simulink subsystem "H175_cathode"  (R2022b)
settings: Solver=VariableStepAuto  StartTime=0.0  StopTime=10.0  RelTol=1e-3
libraries: fl_lib x88, nesl_utility x73, SimscapeFluids_lib x10, slpidlib x2, BraytonCycle_lib x2
(part 1 of 4)
settings Model: Creator=adrian.taveras  LastModifiedBy=adrian.taveras

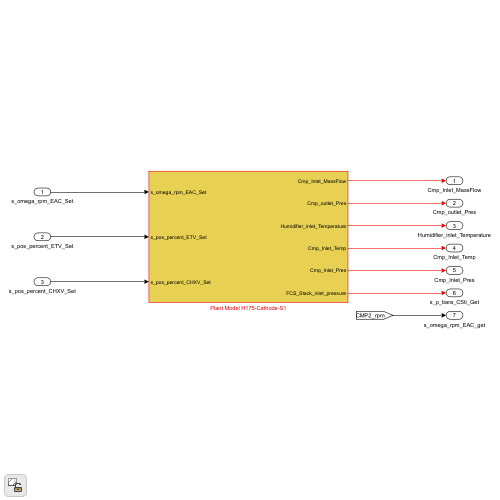
[thumbnail: Simulink's stored preview of the top-level diagram]
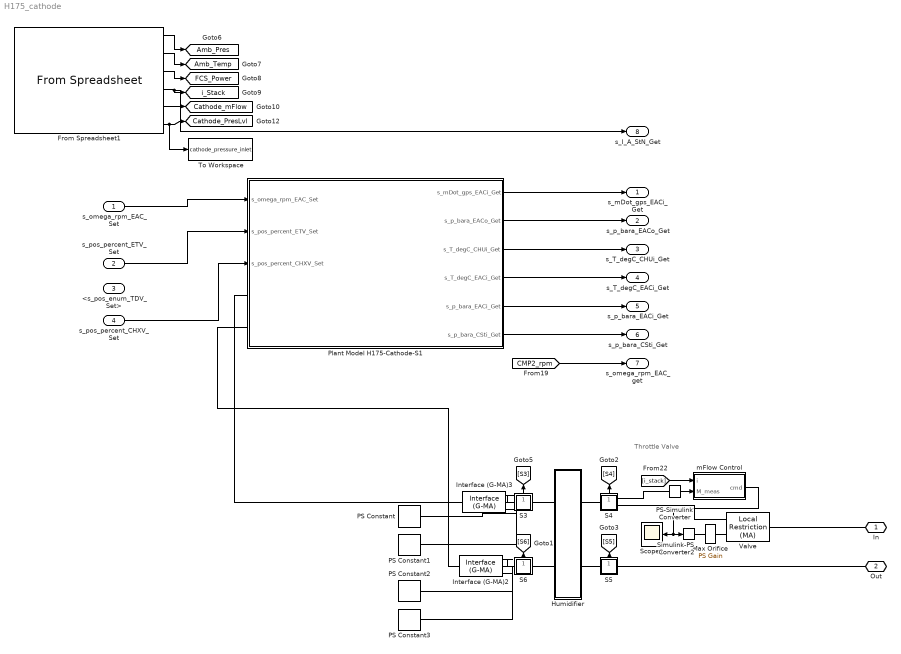
== system H175_cathode ==
  note: Throttle Valve
  s_omega_rpm_EAC_Set : Inport
  s_pos_percent_ETV_Set : Inport  Port=2
  <s_pos_enum_TDV_Set> : Inport  Port=3
  s_pos_percent_CHXV_Set : Inport  Port=4
  From Spreadsheet1 : FromSpreadsheet  FileName=C:\Users\adrian.taveras\Desktop\04-H175-Cathode\H175_Cathode_variables.xlsx  Range=A2:G15
  Humidifier : Subsystem
  Interface (G-MA)2 : SimscapeFluids_lib/Fluid Network Interfaces/Interface (G-MA)  interface_type=foundation.enum.constant_controlled.controlled  moisture_spec=foundation.enum.moisture_spec.relative_humidity  RH_interface=0.5  x_w_interface=0.01  y_w_interface=0.01  HR_interface=0.01  trace_gas_spec=foundation.enum.trace_gas_spec.mass_fraction  x_g_interface=1  y_g_interface=0.001  RH_ws=1  area=0.01 m^2  input_error_spec=foundation.enum.input_range_error.warn
      settings: InternalSimscapePortConfiguration="{\"Bottom\":[{\"id\":\"W\",\"label\":\"W\",\"type\":\"input\"},{\"id\":\"TG\",\"label\":\"TG\",\"type\":\"input\"}],\"Left\":[{\"id\":\"G\",\"label\":\"G\",\"type\":\"foundation.gas.gas\"}],\"Right\":[{\"id\":\"MA\",\"label\":\"MA\",\"type\":\"foundation.moist_air.moist_air\"}],\"Top\":[]}"
  Interface (G-MA)3 : SimscapeFluids_lib/Fluid Network Interfaces/Interface (G-MA)  interface_type=foundation.enum.constant_controlled.controlled  moisture_spec=foundation.enum.moisture_spec.relative_humidity  RH_interface=0.5  x_w_interface=0.01  y_w_interface=0.01  HR_interface=0.01  trace_gas_spec=foundation.enum.trace_gas_spec.mass_fraction  x_g_interface=1  y_g_interface=0.001  RH_ws=1  area=0.01 m^2  input_error_spec=foundation.enum.input_range_error.warn
      settings: InternalSimscapePortConfiguration="{\"Bottom\":[{\"id\":\"W\",\"label\":\"W\",\"type\":\"input\"},{\"id\":\"TG\",\"label\":\"TG\",\"type\":\"input\"}],\"Left\":[{\"id\":\"G\",\"label\":\"G\",\"type\":\"foundation.gas.gas\"}],\"Right\":[{\"id\":\"MA\",\"label\":\"MA\",\"type\":\"foundation.moist_air.moist_air\"}],\"Top\":[]}"
  Max Orifice : fl_lib/Physical Signals/Functions/PS Gain  gain=.008 m^2
  PS Constant : fl_lib/Physical Signals/Sources/PS Constant  constant=.5
  PS Constant1 : fl_lib/Physical Signals/Sources/PS Constant  constant=.001
  PS Constant2 : fl_lib/Physical Signals/Sources/PS Constant  constant=.88
  PS Constant3 : fl_lib/Physical Signals/Sources/PS Constant  constant=.01
  PS-Simulink Converter : nesl_utility/PS-Simulink Converter  PhysicalDomain=network_engine_domain  SubClassName=ps_output  LeftPortType=input  RightPortType=output  PseudoPeriodic=off  Frequencies=[]  VectorFormat=inherit  Unit=inherit  AffineConversion=off
  Plant Model H175-Cathode-S1 : Subsystem
  S3 : Subsystem
      settings: PortSchema="{\"entries\":[{\"content\":{\"sides\":[{\"content\":{\"connectorIds\":[\"LConn1\"]},\"type\":\"ConnectorPlacement.EquallySpacedRectSide\",\"uuid\":\"254e2835-1051-41ce-ae2c-1054ced4b7e5\"},{\"content\":{\"connectorIds\":[\"RConn1\"],\"side\":\"RIGHT\"},\"type\":\"ConnectorPlacement.EquallySpacedRectSide\",\"uuid\":\"319e61c8-525d-4586-8cb8-060a189dde36\"},{\"content\":{\"connectorIds\":[\"Out1\"],\"side\":\"TOP\"},\"type\":\"ConnectorPlacement.EquallySpacedRectSide\",\"uuid\":\"621e15c0-a15c-4528-a2f1-5cf6f15ed99c\"}]},\"type\":\"ConnectorPlacement.EquallySpacedConnector\",\"uuid\":\"0cef8054-f5e2-4319-9020-84a4d4054be4\"}],\"packageUris\":[\"http://schema.mathworks.com/mf0/Connector/R2020b\"],\"version\":\"1.0\"}"
  S4 : Subsystem
      settings: PortSchema="{\"entries\":[{\"content\":{\"sides\":[{\"content\":{\"connectorIds\":[\"LConn1\",\"LConn2\"]},\"type\":\"ConnectorPlacement.EquallySpacedRectSide\",\"uuid\":\"254e2835-1051-41ce-ae2c-1054ced4b7e5\"},{\"content\":{\"connectorIds\":[\"RConn1\"],\"side\":\"RIGHT\"},\"type\":\"ConnectorPlacement.EquallySpacedRectSide\",\"uuid\":\"319e61c8-525d-4586-8cb8-060a189dde36\"},{\"content\":{\"connectorIds\":[\"Out1\"],\"side\":\"TOP\"},\"type\":\"ConnectorPlacement.EquallySpacedRectSide\",\"uuid\":\"621e15c0-a15c-4528-a2f1-5cf6f15ed99c\"}]},\"type\":\"ConnectorPlacement.EquallySpacedConnector\",\"uuid\":\"0cef8054-f5e2-4319-9020-84a4d4054be4\"}],\"packageUris\":[\"http://schema.mathworks.com/mf0/Connector/R2020b\"],\"version\":\"1.0\"}"
  S5 : Subsystem
      settings: PortSchema="{\"entries\":[{\"content\":{\"sides\":[{\"content\":{\"connectorIds\":[\"LConn1\"]},\"type\":\"ConnectorPlacement.EquallySpacedRectSide\",\"uuid\":\"254e2835-1051-41ce-ae2c-1054ced4b7e5\"},{\"content\":{\"connectorIds\":[\"RConn1\"],\"side\":\"RIGHT\"},\"type\":\"ConnectorPlacement.EquallySpacedRectSide\",\"uuid\":\"319e61c8-525d-4586-8cb8-060a189dde36\"},{\"content\":{\"connectorIds\":[\"Out1\"],\"side\":\"TOP\"},\"type\":\"ConnectorPlacement.EquallySpacedRectSide\",\"uuid\":\"621e15c0-a15c-4528-a2f1-5cf6f15ed99c\"},{\"content\":{\"side\":\"BOTTOM\"},\"type\":\"ConnectorPlacement.EquallySpacedRectSide\",\"uuid\":\"5b55ac88-a391-4d8d-b3a5-d7682694097d\"}]},\"type\":\"ConnectorPlacement.EquallySpacedConnector\",\"uuid\":\"0cef8054-f5e2-4319-9020-84a4d4054be4\"}],\"packageUris\":[\"http://schema.mathworks.com/mf0/Connector/R2020b\"],\"version\":\"1.0\"}"
  S6 : Subsystem
      settings: PortSchema="{\"entries\":[{\"content\":{\"sides\":[{\"content\":{\"connectorIds\":[\"LConn1\"]},\"type\":\"ConnectorPlacement.EquallySpacedRectSide\",\"uuid\":\"254e2835-1051-41ce-ae2c-1054ced4b7e5\"},{\"content\":{\"connectorIds\":[\"RConn1\"],\"side\":\"RIGHT\"},\"type\":\"ConnectorPlacement.EquallySpacedRectSide\",\"uuid\":\"319e61c8-525d-4586-8cb8-060a189dde36\"},{\"content\":{\"connectorIds\":[\"Out1\"],\"side\":\"TOP\"},\"type\":\"ConnectorPlacement.EquallySpacedRectSide\",\"uuid\":\"621e15c0-a15c-4528-a2f1-5cf6f15ed99c\"}]},\"type\":\"ConnectorPlacement.EquallySpacedConnector\",\"uuid\":\"0cef8054-f5e2-4319-9020-84a4d4054be4\"}],\"packageUris\":[\"http://schema.mathworks.com/mf0/Connector/R2020b\"],\"version\":\"1.0\"}"
  Scope1 : Scope
  Simulink-PS Converter2 : nesl_utility/Simulink-PS Converter  PhysicalDomain=network_engine_domain  SubClassName=ps_input  LeftPortType=input  RightPortType=output  PseudoPeriodic=off  Frequencies=[]  NoiseDistribution=none  NoiseParameters=[]  Unit=1  AffineConversion=off  FilteringAndDerivatives=filter  SimscapeFilterOrder=1  InputFilterTimeConstant=0.001  UdotUserProvided=0
  To Workspace : ToWorkspace  VariableName=cathode_pressure_inlet  SaveFormat=Timeseries  SampleTime=-1
  Valve : fl_lib/Moist Air/Elements/Local Restriction (MA)  restriction_type=foundation.enum.restriction_type.variable  restriction_area=0.001 m^2  min_area=2e-11 m^2  max_area=.006 m^2  area=.01 m^2  Cd=.64  B_lam=0.999
  mFlow Control : Subsystem
  In : PMIOPort  Side=Left
  Out : PMIOPort  Port=2  Side=Left
  s_mDot_gps_EACi_Get : Outport
  s_p_bara_EACo_Get : Outport  Port=2
  s_T_degC_CHUi_Get : Outport  Port=3
  s_T_degC_EACi_Get : Outport  Port=4
  s_p_bara_EACi_Get : Outport  Port=5
  s_p_bara_CSti_Get : Outport  Port=6
  s_omega_rpm_EAC_get : Outport  Port=7
  s_I_A_StN_Get : Outport  Port=8
  tag scope: Amb_Pres=global, Amb_Temp=global, Cathode_PresLvl=global, Cathode_mFlow=global, FCS_Power=global, i_Stack=global
  wires:
  Plant Model H175-Cathode-S1/3(s_T_degC_CHUi_Get) -> s_T_degC_CHUi_Get/1
  Plant Model H175-Cathode-S1/1(s_mDot_gps_EACi_Get) -> s_mDot_gps_EACi_Get/1
  Plant Model H175-Cathode-S1/2(s_p_bara_EACo_Get) -> s_p_bara_EACo_Get/1
  Plant Model H175-Cathode-S1/4(s_T_degC_EACi_Get) -> s_T_degC_EACi_Get/1
  Plant Model H175-Cathode-S1/5(s_p_bara_EACi_Get) -> s_p_bara_EACi_Get/1
  Plant Model H175-Cathode-S1/6(s_p_bara_CSti_Get) -> s_p_bara_CSti_Get/1
  s_omega_rpm_EAC_Set/1 -> Plant Model H175-Cathode-S1/1(s_omega_rpm_EAC_Set)
  [CMP2_rpm] -> s_omega_rpm_EAC_get/1
  s_pos_percent_ETV_Set/1 -> Plant Model H175-Cathode-S1/2(s_pos_percent_ETV_Set)
  s_pos_percent_CHXV_Set/1 -> Plant Model H175-Cathode-S1/3(s_pos_percent_CHXV_Set)
  From Spreadsheet1/2 -> [Amb_Temp]
  From Spreadsheet1/6 -> [Cathode_PresLvl], To Workspace/1
  From Spreadsheet1/3 -> [FCS_Power]
  From Spreadsheet1/4 -> [i_Stack], s_I_A_StN_Get/1
  From Spreadsheet1/5 -> [Cathode_mFlow]
  From Spreadsheet1/1 -> [Amb_Pres]
  S6/1(Outport) -> [S6]
  S3/1(Outport) -> [S3]
  [i_stack] -> mFlow Control/1(i)
  PS-Simulink Converter/1 -> mFlow Control/2(M_meas)
  mFlow Control/1(cmd) -> Scope1/1, Simulink-PS Converter2/1
  S5/1(Outport) -> [S5]
  S4/1(Outport) -> [S4]
  connections:
  S5/RConn1 -- Humidifier/LConn2
  S3/LConn1 -- Humidifier/RConn1
  Interface (G-MA)3/LConn1 -- Plant Model H175-Cathode-S1/LConn1
  S4/RConn1 -- Humidifier/LConn1
  S4/LConn2 -- Valve/LConn1
  Out/RConn1 -- S5/LConn1
  Simulink-PS Converter2/RConn1 -- Max Orifice/LConn1
  Max Orifice/RConn1 -- Valve/LConn2
  S4/LConn1 -- PS-Simulink Converter/LConn1
  Interface (G-MA)2/RConn1 -- S6/RConn1
  Interface (G-MA)2/LConn1 -- Plant Model H175-Cathode-S1/LConn2
  Valve/RConn1 -- In/RConn1
  Humidifier/RConn2 -- S6/LConn1
  Interface (G-MA)3/RConn1 -- S3/RConn1
  Interface (G-MA)3/RConn2 -- PS Constant/RConn1
  Interface (G-MA)3/RConn3 -- PS Constant1/RConn1
  Interface (G-MA)2/RConn2 -- PS Constant2/RConn1
  Interface (G-MA)2/RConn3 -- PS Constant3/RConn1

== system H175_cathode/Humidifier ==
  Cathode Humidifier1 : Subsystem  Tag=PublishSubsystem
  Cathode Humidifier2 : Subsystem  Tag=PublishSubsystem
  B : PMIOPort  Side=Left
  A1 : PMIOPort  Port=2  Side=Left
  A : PMIOPort  Port=3  Side=Right
  B1 : PMIOPort  Port=4  Side=Right
  connections:
  A1/RConn1 -- Cathode Humidifier2/RConn1
  B/RConn1 -- Cathode Humidifier1/LConn1
  Cathode Humidifier2/LConn1 -- B1/RConn1
  A/RConn1 -- Cathode Humidifier1/RConn1

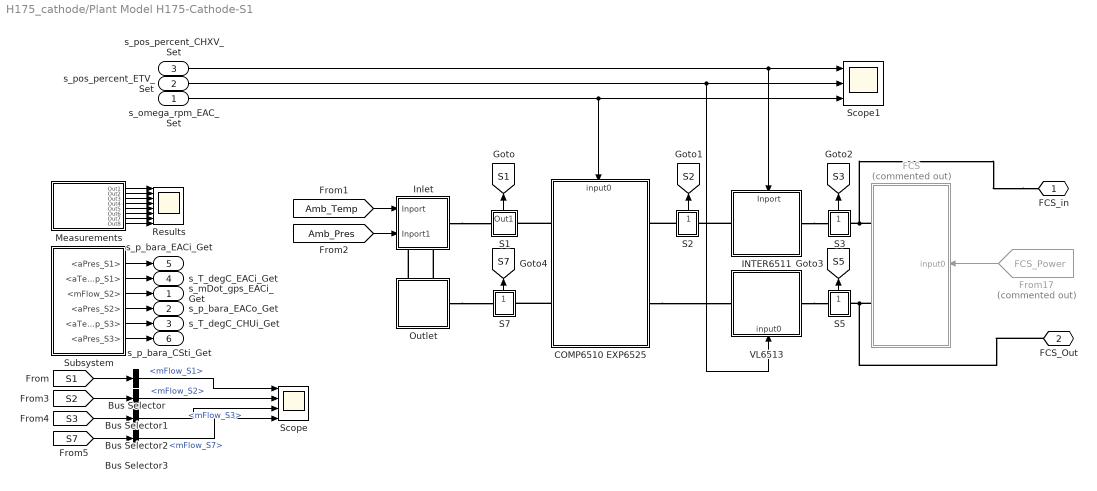
== system H175_cathode/Plant Model H175-Cathode-S1 ==
  s_omega_rpm_EAC_Set : Inport
  s_pos_percent_ETV_Set : Inport  Port=2
  s_pos_percent_CHXV_Set : Inport  Port=3
  "  INTER6511" : Subsystem
      settings: PortSchema="{\"entries\":[{\"content\":{\"sides\":[{\"content\":{\"connectorIds\":[\"LConn1\"]},\"type\":\"ConnectorPlacement.EquallySpacedRectSide\",\"uuid\":\"aadd5cae-df0a-4bff-a962-f45a16973fea\"},{\"content\":{\"connectorIds\":[\"RConn1\"],\"side\":\"RIGHT\"},\"type\":\"ConnectorPlacement.EquallySpacedRectSide\",\"uuid\":\"1cb17e32-c83b-4a61-86cd-0928b2990d84\"},{\"content\":{\"connectorIds\":[\"In1\"],\"side\":\"TOP\"},\"type\":\"ConnectorPlacement.EquallySpacedRectSide\",\"uuid\":\"6373b90c-60a5-4bfd-bcd0-a65342ff5e9d\"}]},\"type\":\"ConnectorPlacement.EquallySpacedConnector\",\"uuid\":\"e3bee535-890d-4344-8b9d-df6658dbcf92\"}],\"packageUris\":[\"http://schema.mathworks.com/mf0/Connector/R2020b\"],\"version\":\"1.0\"}"
  Bus Selector : BusSelector  OutputSignals=mFlow_S1
  Bus Selector1 : BusSelector  OutputSignals=mFlow_S2
  Bus Selector2 : BusSelector  OutputSignals=mFlow_S3
  Bus Selector3 : BusSelector  OutputSignals=mFlow_S7
  COMP6510 EXP6525 : Subsystem
      settings: PortSchema="{\"entries\":[{\"content\":{\"sides\":[{\"content\":{\"connectorIds\":[\"LConn1\",\"LConn2\"]},\"type\":\"ConnectorPlacement.EquallySpacedRectSide\",\"uuid\":\"3b5e743a-f9ab-48a6-a95a-34d49360e365\"},{\"content\":{\"connectorIds\":[\"RConn1\",\"RConn2\"],\"side\":\"RIGHT\"},\"type\":\"ConnectorPlacement.EquallySpacedRectSide\",\"uuid\":\"4725ff20-2386-47e2-9079-da214be67dc0\"},{\"content\":{\"connectorIds\":[\"In1\"],\"side\":\"TOP\"},\"type\":\"ConnectorPlacement.EquallySpacedRectSide\",\"uuid\":\"6967643a-4f8b-418b-b9c8-3e43650ed8fb\"}]},\"type\":\"ConnectorPlacement.EquallySpacedConnector\",\"uuid\":\"78531208-dad3-4e1a-9fde-a0a5eb2a424d\"}],\"packageUris\":[\"http://schema.mathworks.com/mf0/Connector/R2020b\"],\"version\":\"1.0\"}"
  FCS : Subsystem  Commented=on
      settings: PortSchema="{\"entries\":[{\"content\":{\"sides\":[{\"content\":{\"connectorIds\":[\"LConn1\",\"LConn2\"]},\"type\":\"ConnectorPlacement.EquallySpacedRectSide\",\"uuid\":\"2b4fa60d-bbb2-4344-a190-bd8fb686e197\"},{\"content\":{\"connectorIds\":[\"In1\"],\"side\":\"RIGHT\"},\"type\":\"ConnectorPlacement.EquallySpacedRectSide\",\"uuid\":\"0d0ce5e9-3383-4311-ac80-7f18e4d53921\"},{\"content\":{\"connectorIds\":[],\"side\":\"TOP\"},\"type\":\"ConnectorPlacement.EquallySpacedRectSide\",\"uuid\":\"894db579-cef2-48df-a3cf-b374864ac750\"}]},\"type\":\"ConnectorPlacement.EquallySpacedConnector\",\"uuid\":\"d963d44c-ade5-424e-b8d1-081ccbb81476\"}],\"packageUris\":[\"http://schema.mathworks.com/mf0/Connector/R2020b\"],\"version\":\"1.0\"}"
  From17 : From  Commented=on  GotoTag=FCS_Power  TagVisibility=global
  Inlet : Subsystem
      settings: PortSchema="{\"entries\":[{\"content\":{\"sides\":[{\"content\":{\"connectorIds\":[\"In1\",\"In2\"]},\"type\":\"ConnectorPlacement.EquallySpacedRectSide\",\"uuid\":\"383c8b90-d22b-483c-be09-d78d9bde0881\"},{\"content\":{\"connectorIds\":[\"RConn1\"],\"side\":\"RIGHT\"},\"type\":\"ConnectorPlacement.EquallySpacedRectSide\",\"uuid\":\"3dc3e004-4331-4c40-8051-329aa9250422\"},{\"content\":{\"side\":\"TOP\"},\"type\":\"ConnectorPlacement.EquallySpacedRectSide\",\"uuid\":\"aff35d8f-ac03-451a-b72e-dc7bd89924e8\"},{\"content\":{\"connectorIds\":[\"RConn2\",\"RConn3\"],\"side\":\"BOTTOM\"},\"type\":\"ConnectorPlacement.EquallySpacedRectSide\",\"uuid\":\"82493911-a5c4-468a-a003-983b92ffd105\"}]},\"type\":\"ConnectorPlacement.EquallySpacedConnector\",\"uuid\":\"d9a1e9aa-22f5-4e42-bf15-8a8ecd9f58f9\"}],\"packageUris\":[\"http://schema.mathworks.com/mf0/Connector/R2020b\"],\"version\":\"1.0\"}"
  Measurements : Subsystem
  Outlet : Subsystem
      settings: PortSchema="{\"entries\":[{\"content\":{\"sides\":[{\"content\":{\"connectorIds\":[]},\"type\":\"ConnectorPlacement.EquallySpacedRectSide\",\"uuid\":\"36868ebe-cd3e-431e-8c92-72eff994fdca\"},{\"content\":{\"connectorIds\":[\"RConn1\"],\"side\":\"RIGHT\"},\"type\":\"ConnectorPlacement.EquallySpacedRectSide\",\"uuid\":\"888b4745-0282-499a-ac24-9932e912f806\"},{\"content\":{\"connectorIds\":[\"LConn1\",\"LConn2\"],\"side\":\"TOP\"},\"type\":\"ConnectorPlacement.EquallySpacedRectSide\",\"uuid\":\"c9640cda-325e-4343-a4ee-57b72cddf09b\"}]},\"type\":\"ConnectorPlacement.EquallySpacedConnector\",\"uuid\":\"8844a185-194b-4897-895e-d4ee7951df66\"}],\"packageUris\":[\"http://schema.mathworks.com/mf0/Connector/R2020b\"],\"version\":\"1.0\"}"
  Results : Scope  NumInputPorts=8
  S1 : Subsystem
      settings: PortSchema="{\"entries\":[{\"content\":{\"sides\":[{\"content\":{\"connectorIds\":[\"LConn1\"]},\"type\":\"ConnectorPlacement.EquallySpacedRectSide\",\"uuid\":\"872c3fc9-10e2-440a-866c-17ec3b229dcc\"},{\"content\":{\"connectorIds\":[\"RConn1\"],\"side\":\"RIGHT\"},\"type\":\"ConnectorPlacement.EquallySpacedRectSide\",\"uuid\":\"5792e744-d6fd-4953-8a6b-3bc8a25af09f\"},{\"content\":{\"connectorIds\":[\"Out1\"],\"side\":\"TOP\"},\"type\":\"ConnectorPlacement.EquallySpacedRectSide\",\"uuid\":\"2a1362d0-5fde-44c4-8ae5-faebfba0e935\"}]},\"type\":\"ConnectorPlacement.EquallySpacedConnector\",\"uuid\":\"2555ecf8-f6a2-49b2-8cff-d299990cd611\"}],\"packageUris\":[\"http://schema.mathworks.com/mf0/Connector/R2020b\"],\"version\":\"1.0\"}"
  S2 : Subsystem
      settings: PortSchema="{\"entries\":[{\"content\":{\"sides\":[{\"content\":{\"connectorIds\":[\"LConn1\"]},\"type\":\"ConnectorPlacement.EquallySpacedRectSide\",\"uuid\":\"872c3fc9-10e2-440a-866c-17ec3b229dcc\"},{\"content\":{\"connectorIds\":[\"RConn1\"],\"side\":\"RIGHT\"},\"type\":\"ConnectorPlacement.EquallySpacedRectSide\",\"uuid\":\"5792e744-d6fd-4953-8a6b-3bc8a25af09f\"},{\"content\":{\"connectorIds\":[\"Out1\"],\"side\":\"TOP\"},\"type\":\"ConnectorPlacement.EquallySpacedRectSide\",\"uuid\":\"2a1362d0-5fde-44c4-8ae5-faebfba0e935\"}]},\"type\":\"ConnectorPlacement.EquallySpacedConnector\",\"uuid\":\"2555ecf8-f6a2-49b2-8cff-d299990cd611\"}],\"packageUris\":[\"http://schema.mathworks.com/mf0/Connector/R2020b\"],\"version\":\"1.0\"}"
  S3 : Subsystem
      settings: PortSchema="{\"entries\":[{\"content\":{\"sides\":[{\"content\":{\"connectorIds\":[\"LConn1\"]},\"type\":\"ConnectorPlacement.EquallySpacedRectSide\",\"uuid\":\"872c3fc9-10e2-440a-866c-17ec3b229dcc\"},{\"content\":{\"connectorIds\":[\"RConn1\"],\"side\":\"RIGHT\"},\"type\":\"ConnectorPlacement.EquallySpacedRectSide\",\"uuid\":\"5792e744-d6fd-4953-8a6b-3bc8a25af09f\"},{\"content\":{\"connectorIds\":[\"Out1\"],\"side\":\"TOP\"},\"type\":\"ConnectorPlacement.EquallySpacedRectSide\",\"uuid\":\"2a1362d0-5fde-44c4-8ae5-faebfba0e935\"}]},\"type\":\"ConnectorPlacement.EquallySpacedConnector\",\"uuid\":\"2555ecf8-f6a2-49b2-8cff-d299990cd611\"}],\"packageUris\":[\"http://schema.mathworks.com/mf0/Connector/R2020b\"],\"version\":\"1.0\"}"
  S5 : Subsystem
      settings: PortSchema="{\"entries\":[{\"content\":{\"sides\":[{\"content\":{\"connectorIds\":[\"LConn1\"]},\"type\":\"ConnectorPlacement.EquallySpacedRectSide\",\"uuid\":\"872c3fc9-10e2-440a-866c-17ec3b229dcc\"},{\"content\":{\"connectorIds\":[\"RConn1\"],\"side\":\"RIGHT\"},\"type\":\"ConnectorPlacement.EquallySpacedRectSide\",\"uuid\":\"5792e744-d6fd-4953-8a6b-3bc8a25af09f\"},{\"content\":{\"connectorIds\":[\"Out1\"],\"side\":\"TOP\"},\"type\":\"ConnectorPlacement.EquallySpacedRectSide\",\"uuid\":\"2a1362d0-5fde-44c4-8ae5-faebfba0e935\"}]},\"type\":\"ConnectorPlacement.EquallySpacedConnector\",\"uuid\":\"2555ecf8-f6a2-49b2-8cff-d299990cd611\"}],\"packageUris\":[\"http://schema.mathworks.com/mf0/Connector/R2020b\"],\"version\":\"1.0\"}"
  S7 : Subsystem
      settings: PortSchema="{\"entries\":[{\"content\":{\"sides\":[{\"content\":{\"connectorIds\":[\"LConn1\"]},\"type\":\"ConnectorPlacement.EquallySpacedRectSide\",\"uuid\":\"872c3fc9-10e2-440a-866c-17ec3b229dcc\"},{\"content\":{\"connectorIds\":[\"RConn1\"],\"side\":\"RIGHT\"},\"type\":\"ConnectorPlacement.EquallySpacedRectSide\",\"uuid\":\"5792e744-d6fd-4953-8a6b-3bc8a25af09f\"},{\"content\":{\"connectorIds\":[\"Out1\"],\"side\":\"TOP\"},\"type\":\"ConnectorPlacement.EquallySpacedRectSide\",\"uuid\":\"2a1362d0-5fde-44c4-8ae5-faebfba0e935\"}]},\"type\":\"ConnectorPlacement.EquallySpacedConnector\",\"uuid\":\"2555ecf8-f6a2-49b2-8cff-d299990cd611\"}],\"packageUris\":[\"http://schema.mathworks.com/mf0/Connector/R2020b\"],\"version\":\"1.0\"}"
  Scope : Scope  NumInputPorts=4
  Scope1 : Scope  NumInputPorts=3
  Subsystem : Subsystem
  VL6513 : Subsystem
      settings: PortSchema="{\"entries\":[{\"content\":{\"sides\":[{\"content\":{\"connectorIds\":[\"LConn1\"]},\"type\":\"ConnectorPlacement.EquallySpacedRectSide\",\"uuid\":\"aadd5cae-df0a-4bff-a962-f45a16973fea\"},{\"content\":{\"connectorIds\":[\"RConn1\"],\"side\":\"RIGHT\"},\"type\":\"ConnectorPlacement.EquallySpacedRectSide\",\"uuid\":\"1cb17e32-c83b-4a61-86cd-0928b2990d84\"},{\"content\":{\"connectorIds\":[],\"side\":\"TOP\"},\"type\":\"ConnectorPlacement.EquallySpacedRectSide\",\"uuid\":\"6373b90c-60a5-4bfd-bcd0-a65342ff5e9d\"},{\"content\":{\"connectorIds\":[\"In1\"],\"side\":\"BOTTOM\"},\"type\":\"ConnectorPlacement.EquallySpacedRectSide\",\"uuid\":\"d931d881-84c0-4cfd-a67b-0ca607edaec5\"}]},\"type\":\"ConnectorPlacement.EquallySpacedConnector\",\"uuid\":\"e3bee535-890d-4344-8b9d-df6658dbcf92\"}],\"packageUris\":[\"http://schema.mathworks.com/mf0/Connector/R2020b\"],\"version\":\"1.0\"}"
  FCS_in : PMIOPort  Side=Left
  FCS_Out : PMIOPort  Port=2  Side=Left
  s_mDot_gps_EACi_Get : Outport
  s_p_bara_EACo_Get : Outport  Port=2
  s_T_degC_CHUi_Get : Outport  Port=3
  s_T_degC_EACi_Get : Outport  Port=4
  s_p_bara_EACi_Get : Outport  Port=5
  s_p_bara_CSti_Get : Outport  Port=6
  tag scope: S1=global, S2=global, S3=global, S5=global, S7=global
  wires:
  Bus Selector3/1 -> Scope/4  "<mFlow_S7>"
  Bus Selector2/1 -> Scope/3  "<mFlow_S3>"
  Bus Selector1/1 -> Scope/2  "<mFlow_S2>"
  Bus Selector/1 -> Scope/1  "<mFlow_S1>"
  [S7] -> Bus Selector3/1
  [S3] -> Bus Selector2/1
  [S2] -> Bus Selector1/1
  [S1] -> Bus Selector/1
  s_pos_percent_CHXV_Set/1 -> Scope1/1, "  INTER6511"/1(Inport)
  Measurements/8(Out8) -> Results/8
  s_omega_rpm_EAC_Set/1 -> Scope1/3, COMP6510 EXP6525/1(input0)
  Subsystem/4(<aPres_S2>) -> s_p_bara_EACo_Get/1
  Subsystem/2(<aTemp_S1>) -> s_T_degC_EACi_Get/1
  Subsystem/3(<mFlow_S2>) -> s_mDot_gps_EACi_Get/1
  Subsystem/1(<aPres_S1>) -> s_p_bara_EACi_Get/1
  Subsystem/5(<aTemp_S3>) -> s_T_degC_CHUi_Get/1
  Subsystem/6(<aPres_S3>) -> s_p_bara_CSti_Get/1
  S2/1(Out1) -> [S2]
  [Amb_Temp] -> Inlet/1(Inport)
  S7/1(Out1) -> [S7]
  S1/1(Out1) -> [S1]
  [Amb_Pres] -> Inlet/2(Inport1)
  Measurements/6(Out6) -> Results/6
  Measurements/7(Out7) -> Results/7
  Measurements/1(Out1) -> Results/1
  Measurements/3(Out3) -> Results/3
  Measurements/4(Out4) -> Results/4
  Measurements/2(Out2) -> Results/2
  Measurements/5(Out5) -> Results/5
  S3/1(Out1) -> [S3]
  S5/1(Out1) -> [S5]
  s_pos_percent_ETV_Set/1 -> VL6513/1(input0), Scope1/2
  From17/1 -> FCS/1(input0)
  connections:
  COMP6510 EXP6525/RConn2 -- VL6513/LConn1
  COMP6510 EXP6525/LConn2 -- S7/LConn1
  S2/LConn1 -- COMP6510 EXP6525/RConn1
  COMP6510 EXP6525/LConn1 -- S1/RConn1
  "  INTER6511"/LConn1 -- S2/RConn1
  Outlet/LConn2 -- Inlet/RConn3
  Inlet/RConn1 -- S1/LConn1
  Outlet/RConn1 -- S7/RConn1
  Outlet/LConn1 -- Inlet/RConn2
  "  INTER6511"/RConn1 -- S3/RConn1
  FCS_Out/RConn1 -- FCS/LConn2 -- S5/LConn1
  VL6513/RConn1 -- S5/RConn1
  FCS_in/RConn1 -- FCS/LConn1 -- S3/LConn1

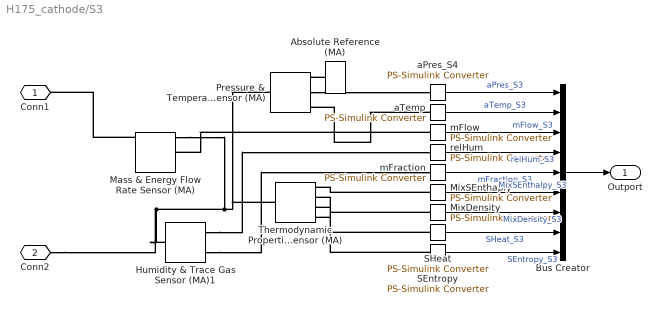
== system H175_cathode/S3 ==
  Absolute Reference (MA) : fl_lib/Moist Air/Elements/Absolute Reference (MA)
  Bus Creator : BusCreator  Inputs=9
  Humidity & Trace Gas Sensor (MA)1 : fl_lib/Moist Air/Sensors/Humidity & Trace Gas Sensor (MA)  moisture_spec=foundation.enum.moisture_spec.relative_humidity  trace_gas_spec=foundation.enum.trace_gas_spec.mass_fraction
      settings: InternalSimscapePortConfiguration="{\"Bottom\":[],\"Left\":[{\"id\":\"A\",\"label\":\"A\",\"type\":\"foundation.moist_air.moist_air\"}],\"Right\":[{\"id\":\"W\",\"label\":\"W\",\"type\":\"output\"},{\"id\":\"G\",\"label\":\"G\",\"type\":\"output\"}],\"Top\":[]}"
  Mass & Energy Flow Rate Sensor (MA) : fl_lib/Moist Air/Sensors/Mass & Energy Flow Rate Sensor (MA)
      settings: InternalSimscapePortConfiguration="{\"Bottom\":[],\"Left\":[{\"id\":\"A\",\"label\":\"A\",\"type\":\"foundation.moist_air.moist_air\"},{\"id\":\"Mw\",\"label\":\"Mw\",\"type\":\"output\"},{\"id\":\"Mg\",\"label\":\"Mg\",\"type\":\"output\"}],\"Right\":[{\"id\":\"B\",\"label\":\"B\",\"type\":\"foundation.moist_air.moist_air\"},{\"id\":\"M\",\"label\":\"M\",\"type\":\"output\"},{\"id\":\"PHI\",\"label\":\"Phi\",\"type\":\"output\"}],\"Top\":[]}"
  MixDensity : nesl_utility/PS-Simulink Converter  PhysicalDomain=network_engine_domain  SubClassName=ps_output  LeftPortType=input  RightPortType=output  PseudoPeriodic=off  Frequencies=[]  VectorFormat=inherit  Unit=inherit  AffineConversion=off
  MixSEnthaply : nesl_utility/PS-Simulink Converter  PhysicalDomain=network_engine_domain  SubClassName=ps_output  LeftPortType=input  RightPortType=output  PseudoPeriodic=off  Frequencies=[]  VectorFormat=inherit  Unit=inherit  AffineConversion=off
  Pressure & Temperature Sensor (MA) : fl_lib/Moist Air/Sensors/Pressure & Temperature Sensor (MA)
      settings: InternalSimscapePortConfiguration="{\"Bottom\":[],\"Left\":[{\"id\":\"A\",\"label\":\"A\",\"type\":\"foundation.moist_air.moist_air\"}],\"Right\":[{\"id\":\"B\",\"label\":\"B\",\"type\":\"foundation.moist_air.moist_air\"},{\"id\":\"P\",\"label\":\"P\",\"type\":\"output\"},{\"id\":\"T\",\"label\":\"T\",\"type\":\"output\"}],\"Top\":[]}"
  SEntropy : nesl_utility/PS-Simulink Converter  PhysicalDomain=network_engine_domain  SubClassName=ps_output  LeftPortType=input  RightPortType=output  PseudoPeriodic=off  Frequencies=[]  VectorFormat=inherit  Unit=inherit  AffineConversion=off
  SHeat : nesl_utility/PS-Simulink Converter  PhysicalDomain=network_engine_domain  SubClassName=ps_output  LeftPortType=input  RightPortType=output  PseudoPeriodic=off  Frequencies=[]  VectorFormat=inherit  Unit=inherit  AffineConversion=off
  Thermodynamic Properties Sensor (MA) : fl_lib/Moist Air/Sensors/Thermodynamic Properties Sensor (MA)  measurement_mass_spec=foundation.enum.measurement_mass_spec.mixture
      settings: InternalSimscapePortConfiguration="{\"Bottom\":[],\"Left\":[{\"id\":\"A\",\"label\":\"A\",\"type\":\"foundation.moist_air.moist_air\"}],\"Right\":[{\"id\":\"H\",\"label\":\"h\",\"type\":\"output\"},{\"id\":\"RHO\",\"label\":\"rho\",\"type\":\"output\"},{\"id\":\"CP\",\"label\":\"cp\",\"type\":\"output\"},{\"id\":\"S\",\"label\":\"s\",\"type\":\"output\"}],\"Top\":[]}"
  aPres_S4 : nesl_utility/PS-Simulink Converter  PhysicalDomain=network_engine_domain  SubClassName=ps_output  LeftPortType=input  RightPortType=output  PseudoPeriodic=off  Frequencies=[]  VectorFormat=inherit  Unit=inherit  AffineConversion=off
  aTemp : nesl_utility/PS-Simulink Converter  PhysicalDomain=network_engine_domain  SubClassName=ps_output  LeftPortType=input  RightPortType=output  PseudoPeriodic=off  Frequencies=[]  VectorFormat=inherit  Unit=inherit  AffineConversion=off
  mFlow : nesl_utility/PS-Simulink Converter  PhysicalDomain=network_engine_domain  SubClassName=ps_output  LeftPortType=input  RightPortType=output  PseudoPeriodic=off  Frequencies=[]  VectorFormat=inherit  Unit=inherit  AffineConversion=off
  mFraction : nesl_utility/PS-Simulink Converter  PhysicalDomain=network_engine_domain  SubClassName=ps_output  LeftPortType=input  RightPortType=output  PseudoPeriodic=off  Frequencies=[]  VectorFormat=inherit  Unit=inherit  AffineConversion=off
  relHum : nesl_utility/PS-Simulink Converter  PhysicalDomain=network_engine_domain  SubClassName=ps_output  LeftPortType=input  RightPortType=output  PseudoPeriodic=off  Frequencies=[]  VectorFormat=inherit  Unit=inherit  AffineConversion=off
  Conn1 : PMIOPort  Side=Left
  Conn2 : PMIOPort  Port=2  Side=Right
  Outport : Outport
  wires:
  SHeat/1 -> Bus Creator/8  "SHeat_S3"
  Bus Creator/1 -> Outport/1
  relHum/1 -> Bus Creator/4  "relHum_S3"
  mFlow/1 -> Bus Creator/3  "mFlow_S3"
  mFraction/1 -> Bus Creator/5  "mFraction_S3"
  MixDensity/1 -> Bus Creator/7  "MixDensity_S3"
  MixSEnthaply/1 -> Bus Creator/6  "MixSEnthalpy_S3"
  SEntropy/1 -> Bus Creator/9  "SEntropy_S3"
  aPres_S4/1 -> Bus Creator/1  "aPres_S3"
  aTemp/1 -> Bus Creator/2  "aTemp_S3"
  connections:
  Absolute Reference (MA)/LConn1 -- Pressure & Temperature Sensor (MA)/RConn1
  Humidity & Trace Gas Sensor (MA)1/RConn2 -- mFraction/LConn1
  Pressure & Temperature Sensor (MA)/RConn2 -- aPres_S4/LConn1
  mFlow/LConn1 -- Mass & Energy Flow Rate Sensor (MA)/RConn2
  Humidity & Trace Gas Sensor (MA)1/LConn1 -- Pressure & Temperature Sensor (MA)/LConn1 -- Thermodynamic Properties Sensor (MA)/LConn1 -- Mass & Energy Flow Rate Sensor (MA)/RConn1 -- Conn2/RConn1
  SEntropy/LConn1 -- Thermodynamic Properties Sensor (MA)/RConn3
  aTemp/LConn1 -- Pressure & Temperature Sensor (MA)/RConn3
  SHeat/LConn1 -- Thermodynamic Properties Sensor (MA)/RConn4
  MixDensity/LConn1 -- Thermodynamic Properties Sensor (MA)/RConn2
  MixSEnthaply/LConn1 -- Thermodynamic Properties Sensor (MA)/RConn1
  Humidity & Trace Gas Sensor (MA)1/RConn1 -- relHum/LConn1
  Mass & Energy Flow Rate Sensor (MA)/LConn1 -- Conn1/RConn1

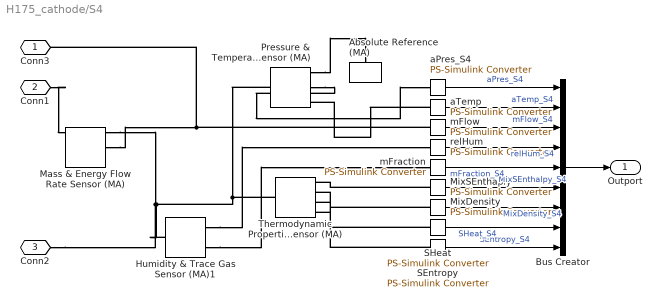
== system H175_cathode/S4 ==
  Absolute Reference (MA) : fl_lib/Moist Air/Elements/Absolute Reference (MA)
  Bus Creator : BusCreator  Inputs=9
  Humidity & Trace Gas Sensor (MA)1 : fl_lib/Moist Air/Sensors/Humidity & Trace Gas Sensor (MA)  moisture_spec=foundation.enum.moisture_spec.relative_humidity  trace_gas_spec=foundation.enum.trace_gas_spec.mass_fraction
      settings: InternalSimscapePortConfiguration="{\"Bottom\":[],\"Left\":[{\"id\":\"A\",\"label\":\"A\",\"type\":\"foundation.moist_air.moist_air\"}],\"Right\":[{\"id\":\"W\",\"label\":\"W\",\"type\":\"output\"},{\"id\":\"G\",\"label\":\"G\",\"type\":\"output\"}],\"Top\":[]}"
  Mass & Energy Flow Rate Sensor (MA) : fl_lib/Moist Air/Sensors/Mass & Energy Flow Rate Sensor (MA)
      settings: InternalSimscapePortConfiguration="{\"Bottom\":[],\"Left\":[{\"id\":\"A\",\"label\":\"A\",\"type\":\"foundation.moist_air.moist_air\"},{\"id\":\"Mw\",\"label\":\"Mw\",\"type\":\"output\"},{\"id\":\"Mg\",\"label\":\"Mg\",\"type\":\"output\"}],\"Right\":[{\"id\":\"B\",\"label\":\"B\",\"type\":\"foundation.moist_air.moist_air\"},{\"id\":\"M\",\"label\":\"M\",\"type\":\"output\"},{\"id\":\"PHI\",\"label\":\"Phi\",\"type\":\"output\"}],\"Top\":[]}"
  MixDensity : nesl_utility/PS-Simulink Converter  PhysicalDomain=network_engine_domain  SubClassName=ps_output  LeftPortType=input  RightPortType=output  PseudoPeriodic=off  Frequencies=[]  VectorFormat=inherit  Unit=inherit  AffineConversion=off
  MixSEnthaply : nesl_utility/PS-Simulink Converter  PhysicalDomain=network_engine_domain  SubClassName=ps_output  LeftPortType=input  RightPortType=output  PseudoPeriodic=off  Frequencies=[]  VectorFormat=inherit  Unit=inherit  AffineConversion=off
  Pressure & Temperature Sensor (MA) : fl_lib/Moist Air/Sensors/Pressure & Temperature Sensor (MA)
      settings: InternalSimscapePortConfiguration="{\"Bottom\":[],\"Left\":[{\"id\":\"A\",\"label\":\"A\",\"type\":\"foundation.moist_air.moist_air\"}],\"Right\":[{\"id\":\"B\",\"label\":\"B\",\"type\":\"foundation.moist_air.moist_air\"},{\"id\":\"P\",\"label\":\"P\",\"type\":\"output\"},{\"id\":\"T\",\"label\":\"T\",\"type\":\"output\"}],\"Top\":[]}"
  SEntropy : nesl_utility/PS-Simulink Converter  PhysicalDomain=network_engine_domain  SubClassName=ps_output  LeftPortType=input  RightPortType=output  PseudoPeriodic=off  Frequencies=[]  VectorFormat=inherit  Unit=inherit  AffineConversion=off
  SHeat : nesl_utility/PS-Simulink Converter  PhysicalDomain=network_engine_domain  SubClassName=ps_output  LeftPortType=input  RightPortType=output  PseudoPeriodic=off  Frequencies=[]  VectorFormat=inherit  Unit=inherit  AffineConversion=off
  Thermodynamic Properties Sensor (MA) : fl_lib/Moist Air/Sensors/Thermodynamic Properties Sensor (MA)  measurement_mass_spec=foundation.enum.measurement_mass_spec.mixture
      settings: InternalSimscapePortConfiguration="{\"Bottom\":[],\"Left\":[{\"id\":\"A\",\"label\":\"A\",\"type\":\"foundation.moist_air.moist_air\"}],\"Right\":[{\"id\":\"H\",\"label\":\"h\",\"type\":\"output\"},{\"id\":\"RHO\",\"label\":\"rho\",\"type\":\"output\"},{\"id\":\"CP\",\"label\":\"cp\",\"type\":\"output\"},{\"id\":\"S\",\"label\":\"s\",\"type\":\"output\"}],\"Top\":[]}"
  aPres_S4 : nesl_utility/PS-Simulink Converter  PhysicalDomain=network_engine_domain  SubClassName=ps_output  LeftPortType=input  RightPortType=output  PseudoPeriodic=off  Frequencies=[]  VectorFormat=inherit  Unit=inherit  AffineConversion=off
  aTemp : nesl_utility/PS-Simulink Converter  PhysicalDomain=network_engine_domain  SubClassName=ps_output  LeftPortType=input  RightPortType=output  PseudoPeriodic=off  Frequencies=[]  VectorFormat=inherit  Unit=inherit  AffineConversion=off
  mFlow : nesl_utility/PS-Simulink Converter  PhysicalDomain=network_engine_domain  SubClassName=ps_output  LeftPortType=input  RightPortType=output  PseudoPeriodic=off  Frequencies=[]  VectorFormat=inherit  Unit=inherit  AffineConversion=off
  mFraction : nesl_utility/PS-Simulink Converter  PhysicalDomain=network_engine_domain  SubClassName=ps_output  LeftPortType=input  RightPortType=output  PseudoPeriodic=off  Frequencies=[]  VectorFormat=inherit  Unit=inherit  AffineConversion=off
  relHum : nesl_utility/PS-Simulink Converter  PhysicalDomain=network_engine_domain  SubClassName=ps_output  LeftPortType=input  RightPortType=output  PseudoPeriodic=off  Frequencies=[]  VectorFormat=inherit  Unit=inherit  AffineConversion=off
  Conn3 : PMIOPort  Side=Left
  Conn1 : PMIOPort  Port=2  Side=Left
  Conn2 : PMIOPort  Port=3  Side=Right
  Outport : Outport
  wires:
  aTemp/1 -> Bus Creator/2  "aTemp_S4"
  aPres_S4/1 -> Bus Creator/1  "aPres_S4"
  SEntropy/1 -> Bus Creator/9  "SEntropy_S4"
  MixSEnthaply/1 -> Bus Creator/6  "MixSEnthalpy_S4"
  MixDensity/1 -> Bus Creator/7  "MixDensity_S4"
  mFraction/1 -> Bus Creator/5  "mFraction_S4"
  mFlow/1 -> Bus Creator/3  "mFlow_S4"
  relHum/1 -> Bus Creator/4  "relHum_S4"
  Bus Creator/1 -> Outport/1
  SHeat/1 -> Bus Creator/8  "SHeat_S4"
  connections:
  Pressure & Temperature Sensor (MA)/RConn1 -- Absolute Reference (MA)/LConn1
  Conn1/RConn1 -- Mass & Energy Flow Rate Sensor (MA)/LConn1
  Humidity & Trace Gas Sensor (MA)1/RConn1 -- relHum/LConn1
  MixSEnthaply/LConn1 -- Thermodynamic Properties Sensor (MA)/RConn1
  MixDensity/LConn1 -- Thermodynamic Properties Sensor (MA)/RConn2
  SHeat/LConn1 -- Thermodynamic Properties Sensor (MA)/RConn4
  aTemp/LConn1 -- Pressure & Temperature Sensor (MA)/RConn3
  SEntropy/LConn1 -- Thermodynamic Properties Sensor (MA)/RConn3
  Humidity & Trace Gas Sensor (MA)1/LConn1 -- Conn2/RConn1 -- Mass & Energy Flow Rate Sensor (MA)/RConn1 -- Thermodynamic Properties Sensor (MA)/LConn1 -- Pressure & Temperature Sensor (MA)/LConn1
  Mass & Energy Flow Rate Sensor (MA)/RConn2 -- Conn3/RConn1 -- mFlow/LConn1
  Pressure & Temperature Sensor (MA)/RConn2 -- aPres_S4/LConn1
  Humidity & Trace Gas Sensor (MA)1/RConn2 -- mFraction/LConn1

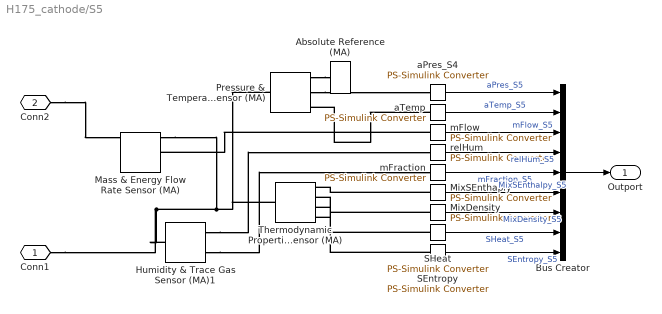
== system H175_cathode/S5 ==
  Absolute Reference (MA) : fl_lib/Moist Air/Elements/Absolute Reference (MA)
  Bus Creator : BusCreator  Inputs=9
  Humidity & Trace Gas Sensor (MA)1 : fl_lib/Moist Air/Sensors/Humidity & Trace Gas Sensor (MA)  moisture_spec=foundation.enum.moisture_spec.relative_humidity  trace_gas_spec=foundation.enum.trace_gas_spec.mass_fraction
      settings: InternalSimscapePortConfiguration="{\"Bottom\":[],\"Left\":[{\"id\":\"A\",\"label\":\"A\",\"type\":\"foundation.moist_air.moist_air\"}],\"Right\":[{\"id\":\"W\",\"label\":\"W\",\"type\":\"output\"},{\"id\":\"G\",\"label\":\"G\",\"type\":\"output\"}],\"Top\":[]}"
  Mass & Energy Flow Rate Sensor (MA) : fl_lib/Moist Air/Sensors/Mass & Energy Flow Rate Sensor (MA)
      settings: InternalSimscapePortConfiguration="{\"Bottom\":[],\"Left\":[{\"id\":\"A\",\"label\":\"A\",\"type\":\"foundation.moist_air.moist_air\"},{\"id\":\"Mw\",\"label\":\"Mw\",\"type\":\"output\"},{\"id\":\"Mg\",\"label\":\"Mg\",\"type\":\"output\"}],\"Right\":[{\"id\":\"B\",\"label\":\"B\",\"type\":\"foundation.moist_air.moist_air\"},{\"id\":\"M\",\"label\":\"M\",\"type\":\"output\"},{\"id\":\"PHI\",\"label\":\"Phi\",\"type\":\"output\"}],\"Top\":[]}"
  MixDensity : nesl_utility/PS-Simulink Converter  PhysicalDomain=network_engine_domain  SubClassName=ps_output  LeftPortType=input  RightPortType=output  PseudoPeriodic=off  Frequencies=[]  VectorFormat=inherit  Unit=inherit  AffineConversion=off
  MixSEnthaply : nesl_utility/PS-Simulink Converter  PhysicalDomain=network_engine_domain  SubClassName=ps_output  LeftPortType=input  RightPortType=output  PseudoPeriodic=off  Frequencies=[]  VectorFormat=inherit  Unit=inherit  AffineConversion=off
  Pressure & Temperature Sensor (MA) : fl_lib/Moist Air/Sensors/Pressure & Temperature Sensor (MA)
      settings: InternalSimscapePortConfiguration="{\"Bottom\":[],\"Left\":[{\"id\":\"A\",\"label\":\"A\",\"type\":\"foundation.moist_air.moist_air\"}],\"Right\":[{\"id\":\"B\",\"label\":\"B\",\"type\":\"foundation.moist_air.moist_air\"},{\"id\":\"P\",\"label\":\"P\",\"type\":\"output\"},{\"id\":\"T\",\"label\":\"T\",\"type\":\"output\"}],\"Top\":[]}"
  SEntropy : nesl_utility/PS-Simulink Converter  PhysicalDomain=network_engine_domain  SubClassName=ps_output  LeftPortType=input  RightPortType=output  PseudoPeriodic=off  Frequencies=[]  VectorFormat=inherit  Unit=inherit  AffineConversion=off
  SHeat : nesl_utility/PS-Simulink Converter  PhysicalDomain=network_engine_domain  SubClassName=ps_output  LeftPortType=input  RightPortType=output  PseudoPeriodic=off  Frequencies=[]  VectorFormat=inherit  Unit=inherit  AffineConversion=off
  Thermodynamic Properties Sensor (MA) : fl_lib/Moist Air/Sensors/Thermodynamic Properties Sensor (MA)  measurement_mass_spec=foundation.enum.measurement_mass_spec.mixture
      settings: InternalSimscapePortConfiguration="{\"Bottom\":[],\"Left\":[{\"id\":\"A\",\"label\":\"A\",\"type\":\"foundation.moist_air.moist_air\"}],\"Right\":[{\"id\":\"H\",\"label\":\"h\",\"type\":\"output\"},{\"id\":\"RHO\",\"label\":\"rho\",\"type\":\"output\"},{\"id\":\"CP\",\"label\":\"cp\",\"type\":\"output\"},{\"id\":\"S\",\"label\":\"s\",\"type\":\"output\"}],\"Top\":[]}"
  aPres_S4 : nesl_utility/PS-Simulink Converter  PhysicalDomain=network_engine_domain  SubClassName=ps_output  LeftPortType=input  RightPortType=output  PseudoPeriodic=off  Frequencies=[]  VectorFormat=inherit  Unit=inherit  AffineConversion=off
  aTemp : nesl_utility/PS-Simulink Converter  PhysicalDomain=network_engine_domain  SubClassName=ps_output  LeftPortType=input  RightPortType=output  PseudoPeriodic=off  Frequencies=[]  VectorFormat=inherit  Unit=inherit  AffineConversion=off
  mFlow : nesl_utility/PS-Simulink Converter  PhysicalDomain=network_engine_domain  SubClassName=ps_output  LeftPortType=input  RightPortType=output  PseudoPeriodic=off  Frequencies=[]  VectorFormat=inherit  Unit=inherit  AffineConversion=off
  mFraction : nesl_utility/PS-Simulink Converter  PhysicalDomain=network_engine_domain  SubClassName=ps_output  LeftPortType=input  RightPortType=output  PseudoPeriodic=off  Frequencies=[]  VectorFormat=inherit  Unit=inherit  AffineConversion=off
  relHum : nesl_utility/PS-Simulink Converter  PhysicalDomain=network_engine_domain  SubClassName=ps_output  LeftPortType=input  RightPortType=output  PseudoPeriodic=off  Frequencies=[]  VectorFormat=inherit  Unit=inherit  AffineConversion=off
  Conn1 : PMIOPort  Side=Left
  Conn2 : PMIOPort  Port=2  Side=Right
  Outport : Outport
  wires:
  SHeat/1 -> Bus Creator/8  "SHeat_S5"
  Bus Creator/1 -> Outport/1
  relHum/1 -> Bus Creator/4  "relHum_S5"
  mFlow/1 -> Bus Creator/3  "mFlow_S5"
  mFraction/1 -> Bus Creator/5  "mFraction_S5"
  MixDensity/1 -> Bus Creator/7  "MixDensity_S5"
  MixSEnthaply/1 -> Bus Creator/6  "MixSEnthalpy_S5"
  SEntropy/1 -> Bus Creator/9  "SEntropy_S5"
  aPres_S4/1 -> Bus Creator/1  "aPres_S5"
  aTemp/1 -> Bus Creator/2  "aTemp_S5"
  connections:
  Pressure & Temperature Sensor (MA)/RConn1 -- Absolute Reference (MA)/LConn1
  Humidity & Trace Gas Sensor (MA)1/RConn2 -- mFraction/LConn1
  Pressure & Temperature Sensor (MA)/RConn2 -- aPres_S4/LConn1
  mFlow/LConn1 -- Mass & Energy Flow Rate Sensor (MA)/RConn2
  Humidity & Trace Gas Sensor (MA)1/LConn1 -- Pressure & Temperature Sensor (MA)/LConn1 -- Thermodynamic Properties Sensor (MA)/LConn1 -- Mass & Energy Flow Rate Sensor (MA)/RConn1 -- Conn1/RConn1
  SEntropy/LConn1 -- Thermodynamic Properties Sensor (MA)/RConn3
  aTemp/LConn1 -- Pressure & Temperature Sensor (MA)/RConn3
  SHeat/LConn1 -- Thermodynamic Properties Sensor (MA)/RConn4
  MixDensity/LConn1 -- Thermodynamic Properties Sensor (MA)/RConn2
  MixSEnthaply/LConn1 -- Thermodynamic Properties Sensor (MA)/RConn1
  Humidity & Trace Gas Sensor (MA)1/RConn1 -- relHum/LConn1
  Conn2/RConn1 -- Mass & Energy Flow Rate Sensor (MA)/LConn1

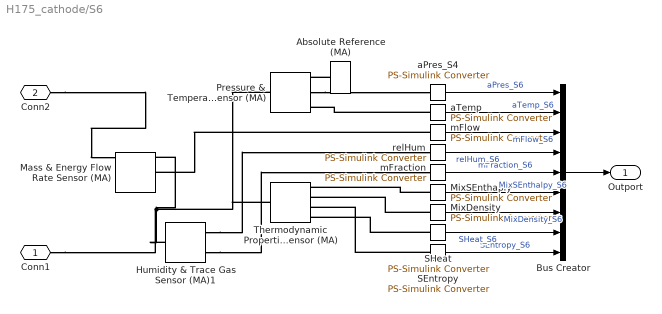
== system H175_cathode/S6 ==
  Absolute Reference (MA) : fl_lib/Moist Air/Elements/Absolute Reference (MA)
  Bus Creator : BusCreator  Inputs=9
  Humidity & Trace Gas Sensor (MA)1 : fl_lib/Moist Air/Sensors/Humidity & Trace Gas Sensor (MA)  moisture_spec=foundation.enum.moisture_spec.relative_humidity  trace_gas_spec=foundation.enum.trace_gas_spec.mass_fraction
      settings: InternalSimscapePortConfiguration="{\"Bottom\":[],\"Left\":[{\"id\":\"A\",\"label\":\"A\",\"type\":\"foundation.moist_air.moist_air\"}],\"Right\":[{\"id\":\"W\",\"label\":\"W\",\"type\":\"output\"},{\"id\":\"G\",\"label\":\"G\",\"type\":\"output\"}],\"Top\":[]}"
  Mass & Energy Flow Rate Sensor (MA) : fl_lib/Moist Air/Sensors/Mass & Energy Flow Rate Sensor (MA)
      settings: InternalSimscapePortConfiguration="{\"Bottom\":[],\"Left\":[{\"id\":\"A\",\"label\":\"A\",\"type\":\"foundation.moist_air.moist_air\"},{\"id\":\"Mw\",\"label\":\"Mw\",\"type\":\"output\"},{\"id\":\"Mg\",\"label\":\"Mg\",\"type\":\"output\"}],\"Right\":[{\"id\":\"B\",\"label\":\"B\",\"type\":\"foundation.moist_air.moist_air\"},{\"id\":\"M\",\"label\":\"M\",\"type\":\"output\"},{\"id\":\"PHI\",\"label\":\"Phi\",\"type\":\"output\"}],\"Top\":[]}"
  MixDensity : nesl_utility/PS-Simulink Converter  PhysicalDomain=network_engine_domain  SubClassName=ps_output  LeftPortType=input  RightPortType=output  PseudoPeriodic=off  Frequencies=[]  VectorFormat=inherit  Unit=inherit  AffineConversion=off
  MixSEnthaply : nesl_utility/PS-Simulink Converter  PhysicalDomain=network_engine_domain  SubClassName=ps_output  LeftPortType=input  RightPortType=output  PseudoPeriodic=off  Frequencies=[]  VectorFormat=inherit  Unit=inherit  AffineConversion=off
  Pressure & Temperature Sensor (MA) : fl_lib/Moist Air/Sensors/Pressure & Temperature Sensor (MA)
      settings: InternalSimscapePortConfiguration="{\"Bottom\":[],\"Left\":[{\"id\":\"A\",\"label\":\"A\",\"type\":\"foundation.moist_air.moist_air\"}],\"Right\":[{\"id\":\"B\",\"label\":\"B\",\"type\":\"foundation.moist_air.moist_air\"},{\"id\":\"P\",\"label\":\"P\",\"type\":\"output\"},{\"id\":\"T\",\"label\":\"T\",\"type\":\"output\"}],\"Top\":[]}"
  SEntropy : nesl_utility/PS-Simulink Converter  PhysicalDomain=network_engine_domain  SubClassName=ps_output  LeftPortType=input  RightPortType=output  PseudoPeriodic=off  Frequencies=[]  VectorFormat=inherit  Unit=inherit  AffineConversion=off
  SHeat : nesl_utility/PS-Simulink Converter  PhysicalDomain=network_engine_domain  SubClassName=ps_output  LeftPortType=input  RightPortType=output  PseudoPeriodic=off  Frequencies=[]  VectorFormat=inherit  Unit=inherit  AffineConversion=off
  Thermodynamic Properties Sensor (MA) : fl_lib/Moist Air/Sensors/Thermodynamic Properties Sensor (MA)  measurement_mass_spec=foundation.enum.measurement_mass_spec.mixture
      settings: InternalSimscapePortConfiguration="{\"Bottom\":[],\"Left\":[{\"id\":\"A\",\"label\":\"A\",\"type\":\"foundation.moist_air.moist_air\"}],\"Right\":[{\"id\":\"H\",\"label\":\"h\",\"type\":\"output\"},{\"id\":\"RHO\",\"label\":\"rho\",\"type\":\"output\"},{\"id\":\"CP\",\"label\":\"cp\",\"type\":\"output\"},{\"id\":\"S\",\"label\":\"s\",\"type\":\"output\"}],\"Top\":[]}"
  aPres_S4 : nesl_utility/PS-Simulink Converter  PhysicalDomain=network_engine_domain  SubClassName=ps_output  LeftPortType=input  RightPortType=output  PseudoPeriodic=off  Frequencies=[]  VectorFormat=inherit  Unit=inherit  AffineConversion=off
  aTemp : nesl_utility/PS-Simulink Converter  PhysicalDomain=network_engine_domain  SubClassName=ps_output  LeftPortType=input  RightPortType=output  PseudoPeriodic=off  Frequencies=[]  VectorFormat=inherit  Unit=inherit  AffineConversion=off
  mFlow : nesl_utility/PS-Simulink Converter  PhysicalDomain=network_engine_domain  SubClassName=ps_output  LeftPortType=input  RightPortType=output  PseudoPeriodic=off  Frequencies=[]  VectorFormat=inherit  Unit=inherit  AffineConversion=off
  mFraction : nesl_utility/PS-Simulink Converter  PhysicalDomain=network_engine_domain  SubClassName=ps_output  LeftPortType=input  RightPortType=output  PseudoPeriodic=off  Frequencies=[]  VectorFormat=inherit  Unit=inherit  AffineConversion=off
  relHum : nesl_utility/PS-Simulink Converter  PhysicalDomain=network_engine_domain  SubClassName=ps_output  LeftPortType=input  RightPortType=output  PseudoPeriodic=off  Frequencies=[]  VectorFormat=inherit  Unit=inherit  AffineConversion=off
  Conn1 : PMIOPort  Side=Left
  Conn2 : PMIOPort  Port=2  Side=Right
  Outport : Outport
  wires:
  aTemp/1 -> Bus Creator/2  "aTemp_S6"
  aPres_S4/1 -> Bus Creator/1  "aPres_S6"
  SEntropy/1 -> Bus Creator/9  "SEntropy_S6"
  MixSEnthaply/1 -> Bus Creator/6  "MixSEnthalpy_S6"
  MixDensity/1 -> Bus Creator/7  "MixDensity_S6"
  mFraction/1 -> Bus Creator/5  "mFraction_S6"
  mFlow/1 -> Bus Creator/3  "mFlow_S6"
  relHum/1 -> Bus Creator/4  "relHum_S6"
  Bus Creator/1 -> Outport/1
  SHeat/1 -> Bus Creator/8  "SHeat_S6"
  connections:
  Absolute Reference (MA)/LConn1 -- Pressure & Temperature Sensor (MA)/RConn1
  Humidity & Trace Gas Sensor (MA)1/LConn1 -- Thermodynamic Properties Sensor (MA)/LConn1 -- Pressure & Temperature Sensor (MA)/LConn1 -- Conn1/RConn1 -- Mass & Energy Flow Rate Sensor (MA)/RConn1
  Humidity & Trace Gas Sensor (MA)1/RConn1 -- relHum/LConn1
  MixSEnthaply/LConn1 -- Thermodynamic Properties Sensor (MA)/RConn1
  MixDensity/LConn1 -- Thermodynamic Properties Sensor (MA)/RConn2
  SHeat/LConn1 -- Thermodynamic Properties Sensor (MA)/RConn4
  aTemp/LConn1 -- Pressure & Temperature Sensor (MA)/RConn3
  SEntropy/LConn1 -- Thermodynamic Properties Sensor (MA)/RConn3
  Conn2/RConn1 -- Mass & Energy Flow Rate Sensor (MA)/LConn1
  mFlow/LConn1 -- Mass & Energy Flow Rate Sensor (MA)/RConn2
  Pressure & Temperature Sensor (MA)/RConn2 -- aPres_S4/LConn1
  Humidity & Trace Gas Sensor (MA)1/RConn2 -- mFraction/LConn1

== system H175_cathode/mFlow Control ==
  i : Inport
  M_meas : Inport  Port=2
  1-D Lookup Table : Lookup_n-D  Commented=on  NumberOfTableDimensions=1  BreakpointsForDimension1=[0;15;20;45;100;200;300;350;400;420;450;500;550;600]  Table=[0;.007;.009;.019;.035;.070;.101;.118;.134;.141;.151;.168;.185;.202]  InterpMethod=Cubic spline  InternalRulePriority=Speed  RndMeth=Simplest
  Constant : Constant  Value=.167
  Control Signals : Scope  NumInputPorts=2
  Gain : Gain  Commented=on  Gain=3.
  Mux : Mux  Inputs=2
  Mux1 : Mux  Inputs=2
  PID Controller1 : slpidlib/PID Controller  Controller=PI  Form=Parallel  TimeDomain=Continuous-time  UseExternalTs=off  SampleTime=-1  IntegratorMethod=Forward Euler  FilterMethod=Forward Euler  ControllerParametersSource=internal  P=49.21  I=6.2008  UseKiTs=off  D=20  N=10  UseFilter=on  TunerSelectOption=Transfer Function Based (PID Tuner App)  InitialConditionSource=internal  InitialConditionForIntegrator=0  InitialConditionForFilter=0  DifferentiatorICPrevScaledInput=0  ExternalReset=none  TrackingMode=off  Kt=1  LimitOutput=on  SatLimitsSource=internal  UpperSaturationLimit=1  LowerSaturationLimit=-1  LinearizeAsGain=off  AntiWindupMode=clamping  Kb=1  LimitIntegrator=off  UpperIntegratorSaturationLimit=inf  LowerIntegratorSaturationLimit=-inf  POutMin=[]  POutMax=[]  IOutMin=[]  IOutMax=[]  DOutMin=[]  DOutMax=[]  NOutMin=[]  NOutMax=[]  SumOutMin=[]  SumOutMax=[]  SaturationOutMin=[]  SaturationOutMax=[]  PParamMin=[]  PParamMax=[]  IParamMin=[]  IParamMax=[]  DParamMin=[]  DParamMax=[]  NParamMin=[]  NParamMax=[]  KbParamMin=[]  KbParamMax=[]  KtParamMin=[]  KtParamMax=[]  KbOutMin=[]  KbOutMax=[]  KtOutMin=[]  KtOutMax=[]  IntegratorOutMin=[]  IntegratorOutMax=[]  FilterOutMin=[]  FilterOutMax=[]  SumI1OutMin=[]  SumI1OutMax=[]  SumI2OutMin=[]  SumI2OutMax=[]  SumI3OutMin=[]  SumI3OutMax=[]  SumI4OutMin=[]  SumI4OutMax=[]  SumDOutMin=[]  SumDOutMax=[]  DifferentiatorOutMin=[]  DifferentiatorOutMax=[]  FilterDiffOutCoefMin=[]  FilterDiffOutCoefMax=[]  ReciprocalOutMin=[]  ReciprocalOutMax=[]  SumDenOutMin=[]  SumDenOutMax=[]  SumNumOutMin=[]  SumNumOutMax=[]  DivideOutMin=[]  DivideOutMax=[]  UdiffTsProdOutMin=[]  UdiffTsProdOutMax=[]  NTsProdOutMin=[]  NTsProdOutMax=[]  UintegralTsProdOutMin=[]  UintegralTsProdOutMax=[]  UngainTsProdOutMin=[]  UngainTsProdOutMax=[]  ClampingZeroOutDataTypeStr=Inherit: Inherit via back propagation  ClampingZeroOutMin=[]  ClampingZeroOutMax=[]  FilterDenConstantOutDataTypeStr=Inherit: Inherit via back propagation  FilterDenConstantOutMin=[]  FilterDenConstantOutMax=[]  PCopyOutDataTypeStr=Inherit: Inherit via back propagation  PCopyOutMin=[]  PCopyOutMax=[]  NCopyOutDataTypeStr=Inherit: Inherit via back propagation  NCopyOutMin=[]  NCopyOutMax=[]  IntegratorContinuousStateAttributes=''  IntegratorStateMustResolveToSignalObject=off  IntegratorRTWStateStorageClass=Auto  FilterContinuousStateAttributes=''  FilterStateMustResolveToSignalObject=off  FilterRTWStateStorageClass=Auto  ParallelPVariant=InternalParameters  IdealPVariant=Disabled  IVariant=InternalParameters  DVariant=Disabled  IntegratorVariant=Continuous  SatVariant=Enabled  AWVariant=ContClampingParallel  PCopyVariant=Disabled  TRVariant=Disabled  FdbkBlocksVariant=Forward  IdealPFdbkVariant=Disabled  SatFdbkVariant=Disabled  DerivativeFilterVariant=Disabled  NVariant=Disabled  NCopyVariant=Disabled_SignalSpec  FilterICVariant=Disabled  IntegratorICVariant=InternalICs  ExternalResetVariant=Disabled  TRSumVariant=Passthrough  SumFdbkVariant=Disabled  SumVariant=Sum_PI  TsampFilterVariant=InternalTs  TsampNgainVariant=Passthrough  TsampIntegralVariant=Passthrough  ExternalSaturationOutDataTypeStr=Inherit: Same as second input
  Sum : Sum  Inputs=|+-
  Transfer Fcn : TransferFcn  Denominator=[1 1]
  cmd : Outport
  wires:
  Gain/1 -> 1-D Lookup Table/1
  Mux1/1 -> Control Signals/2
  Mux/1 -> Control Signals/1
  Transfer Fcn/1 -> cmd/1, Mux1/2
  M_meas/1 -> Sum/2, Mux/2
  Constant/1 -> Mux/1, Sum/1
  Sum/1 -> PID Controller1/1
  PID Controller1/1 -> Transfer Fcn/1, Mux1/1
  i/1 -> Gain/1
